simulink model "example_Hydraulic_PumpConst"  (R2018b)
settings: Solver=ode45  StartTime=0.0  StopTime=240  MaxStep=10  RelTol=1e-3  EnableMultiTasking=on
libraries: carnot x4
settings Model: Creator=drhf  LastModifiedBy=drhf
settings DataIOCC: LimitDataPoints=on  SaveFormat=Array
settings OptimizationCC: ExpressionDepthLimit=2147483647  LifeSpan=inf
settings DebuggingCC: UnderspecifiedInitializationDetection=Classic  MergeDetectMultiDrivingBlocksExec=none  SolverPrmCheckMsg=warning  StateNameClashWarn=warning  SFUnexpectedBacktrackingDiag=warning  SFNoUnconditionalDefaultTransitionDiag=warning  SFExecutionAtInitializationDiag=none
settings HardwareCC: ProdBitPerPointer=32  ProdBitPerSizeT=32  ProdBitPerPtrDiffT=32  ProdLargestAtomicFloat=None  ProdIntDivRoundTo=Undefined  ProdEndianess=Unspecified  ProdWordSize=32  ProdHWDeviceType=32-bit Generic
settings ModelReferenceCC: PropagateSignalLabelsOutOfModel=off
settings SFSimCC: SimUseLocalCustomCode=off
settings RTWCC: RTWUseLocalCustomCode=off
settings CodeAppCC: StateflowObjectComments=on
settings GRTTargetCC: TargetLangStandard=C89/C90 (ANSI)  GeneratePreprocessorConditionals=Disable all  CombineOutputUpdateFcns=off  GRTInterface=on
settings ConfigComp: CovMetricSettings=dw  CovHtmlReporting=on  CovSaveCumulativeToWorkspaceVar=on  CovSaveSingleToWorkspaceVar=on  CovExternalEMLEnable=off

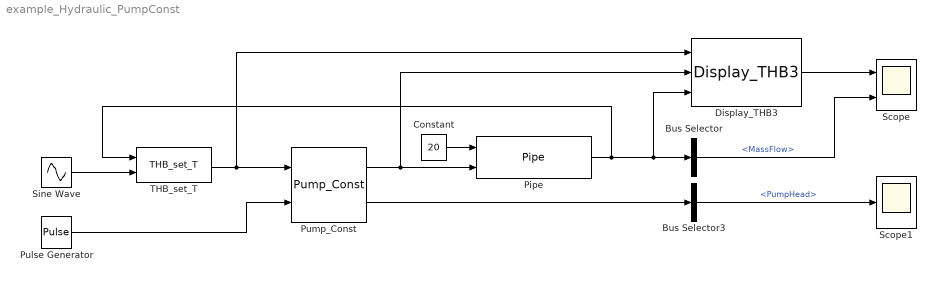
== system example_Hydraulic_PumpConst ==
  Bus Selector : BusSelector  OutputSignals=MassFlow
  Bus Selector3 : BusSelector  OutputSignals=PumpHead
  Constant : Constant  Value=20
  Display_THB3 : carnot/Outputs/Display_THB3  t=on  m=off  p=off  id=off  mix=off  d=off
      settings: SourceProductName=Carnot
  Pipe : carnot/Hydraulics/Pipe  dia=0.02  len=10  hgt=5  uloss=100/20/10  cond=0  cwall=1000  t0=20  lin=100/0.2  qua=100/0.2^2  nodes=10
      settings: SourceProductName=Carnot
  Pulse Generator : DiscretePulseGenerator  PulseType=Time based  Period=100  PulseWidth=50  PhaseDelay=20
  Pump_Const : carnot/Hydraulics/Pump_Const  mdotmax=1200/3600  dia=0.025  p0=3e5  fluid_id=Water  mix=0  mix2=0  mix3=0  UA=1  mcp=2000  Tini=10  e0=10  e1=10  e2=-1
      settings: SourceProductName=Carnot
  Scope : Scope  NumInputPorts=2
  Scope1 : Scope
  Sine Wave : Sin  Amplitude=5  Bias=20  Frequency=2*pi/240  SampleTime=0
  THB_set_T : carnot/Source/Simple/THB_set_T
      settings: SourceProductName=Carnot
  wires:
  Pipe/1 -> Display_THB3/3, Bus Selector/1, THB_set_T/1
  THB_set_T/1 -> Display_THB3/1, Pump_Const/1
  Pulse Generator/1 -> Pump_Const/2
  Pump_Const/2 -> Bus Selector3/1
  Bus Selector/1 -> Scope/2  "<MassFlow>"
  Display_THB3/1 -> Scope/1
  Sine Wave/1 -> THB_set_T/2
  Pump_Const/1 -> Display_THB3/2, Pipe/2
  Constant/1 -> Pipe/1
  Bus Selector3/1 -> Scope1/1  "<PumpHead>"
